simulink model "Simulink_model"  (R2024b)
settings: Solver=VariableStepAuto  StartTime=0.0  StopTime=10.0  RelTol=1e-3
values from neighbouring files (symbols this model uses):
  Gamma_obs = [Gamma, L]    [Script.m]
  H_obs = eye(n)    [Script.m]
  J_obs = zeros(n, m+p)    [Script.m]
  K = place(Phi, Gamma, p_d)    [Script.m]
  Nu = sol(n+1 : end)    [Script.m]
  Nx = sol(1 : n)    [Script.m]
  P_c = 90 / (s^2 + 60*s + 3)    [Script.m]
  Phi_obs = Phi - L*H    [Script.m]
  Ts = Ts_max / 4    (= 0.0218166156499)    [Script.m]
settings Model: Creator=andre  LastModifiedBy=Enrico 2

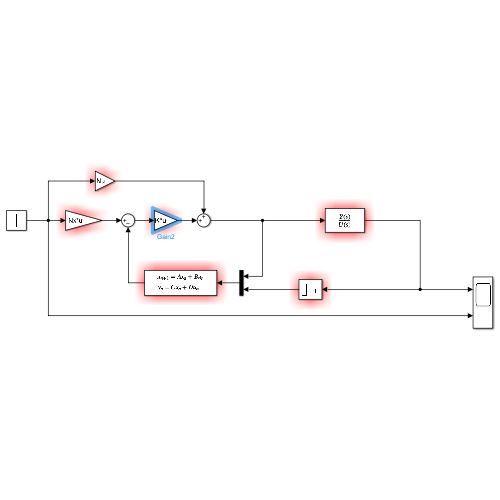
[thumbnail: Simulink's stored preview of the top-level diagram]
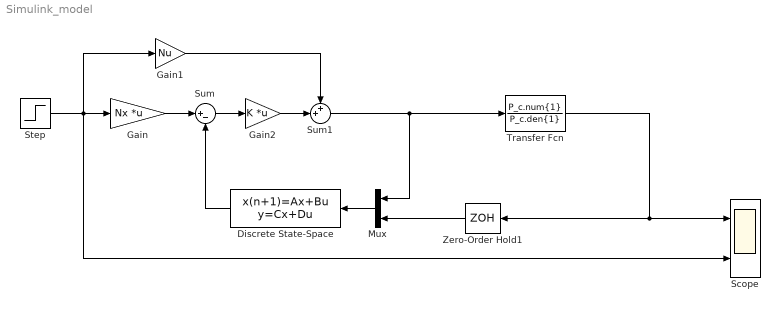
== system Simulink_model ==
  Discrete State-Space : DiscreteStateSpace  A=Phi_obs  B=Gamma_obs  C=H_obs  D=J_obs  SampleTime=Ts
  Gain : Gain  Gain=Nx  Multiplication=Matrix(K*u)
  Gain1 : Gain  Gain=Nu
  Gain2 : Gain  Gain=K  Multiplication=Matrix(K*u)
  Mux : Mux  Inputs=2
  Scope : Scope  NumInputPorts=2
  Step : Step  After=100  SampleTime=0
  Sum : Sum  Inputs=|+-
  Sum1 : Sum  Inputs=++|
  Transfer Fcn : TransferFcn  Numerator=P_c.num{1}  Denominator=P_c.den{1}
  Zero-Order Hold1 : ZeroOrderHold  SampleTime=Ts
  wires:
  Transfer Fcn/1 -> Scope/1, Zero-Order Hold1/1
  Zero-Order Hold1/1 -> Mux/2
  Mux/1 -> Discrete State-Space/1
  Sum1/1 -> Transfer Fcn/1, Mux/1
  Sum/1 -> Gain2/1
  Step/1 -> Scope/2, Gain1/1, Gain/1
  Gain1/1 -> Sum1/1
  Gain/1 -> Sum/1
  Gain2/1 -> Sum1/2
  Discrete State-Space/1 -> Sum/2
